simulink model "BaseEngineController_LS_128"  (Simulink 7.7)
settings: Solver=FixedStepDiscrete  StartTime=0.0  StopTime=10.0  RelTol=1e-3
PreLoadFcn:
  | try, eval([bdroot '_setup']); catch, eval('model_setup', ''); end
InitFcn:
  | try, eval([bdroot '_setup']); catch, eval('model_setup', ''); end
undefined symbols (not defined in the file): ECU565, High, motohawk_build_version, motohawk_trunc_name, motohawk_vardec_config_group, motohawk_vardec_path, True
libraries: MotoHawk_lib x1418, motohawk_control_primitives_lib x183, motohawk_engine_lib x32, simulink x21, motohawk_annotations_lib x9, AutoDoc_lib x8, simulink_extras x4, motohawk_ccp_examples_lib x1, motohawk_control_primitives_motoshare_lib x1
(part 23 of 27)

== system BaseEngineController_LS_128/Foreground/Control/Controller/Run/O2 Control/O2 PID Calibrations ==
  Sensors : Inport
  Bus Creator : BusCreator  Inputs=12
  Error Gain Scheduling : Subsystem
  O2 Control Switch Point Maps : Subsystem
  motohawk_calibration10 : MotoHawk_lib/Calibration & Probing Blocks/motohawk_calibration  nam='O2CtrlPIDOutUpperLimit'  val=10  storage=Calibration  show_more=on  name_source=Use Parameter  data_type=Inherit from 'Default Value'  read_level=1  write_level=1  ovr_cals=on  view_as=Number  enum_struct={'Disabled', 'Enabled'}  vector_style=Wide Row  use_help_units=on  help='Upper limit on gaseous closed loop O2 PID Output.'  units='mult'  use_header_enum=off  row_header_enum={}  col_header_enum={}  use_min_max=off  min_val=-inf  max_val=inf  use_precision=off  precision='5.3'  gain=1  offset=0  exp=1  use_mototune_group=on  mototune_group=motohawk_vardec_path(gcb)
  motohawk_calibration11 : MotoHawk_lib/Calibration & Probing Blocks/motohawk_calibration  nam='O2CtrlPIDOutLowerLimit'  val=-10  storage=Calibration  show_more=on  name_source=Use Parameter  data_type=Inherit from 'Default Value'  read_level=1  write_level=1  ovr_cals=on  view_as=Number  enum_struct={'Disabled', 'Enabled'}  vector_style=Wide Row  use_help_units=on  help='Lower limit on gaseous closed loop O2 PID Output.'  units='mult'  use_header_enum=off  row_header_enum={}  col_header_enum={}  use_min_max=off  min_val=-inf  max_val=inf  use_precision=off  precision='5.3'  gain=1  offset=0  exp=1  use_mototune_group=on  mototune_group=motohawk_vardec_path(gcb)
  motohawk_calibration5 : MotoHawk_lib/Calibration & Probing Blocks/motohawk_calibration  nam='O2CtrlPGain'  val=1  storage=Calibration  show_more=on  name_source=Use Parameter  data_type=Inherit from 'Default Value'  read_level=1  write_level=1  ovr_cals=on  view_as=Number  enum_struct={'Disabled', 'Enabled'}  vector_style=Wide Row  use_help_units=on  help='Base P-gain for the gaseous closed loop O2 controller.'  units='mult'  use_header_enum=off  row_header_enum={}  col_header_enum={}  use_min_max=off  min_val=-inf  max_val=inf  use_precision=off  precision='5.3'  gain=1  offset=0  exp=1  use_mototune_group=on  mototune_group=motohawk_vardec_path(gcb)
  motohawk_calibration6 : MotoHawk_lib/Calibration & Probing Blocks/motohawk_calibration  nam='O2CtrlIGain'  val=1  storage=Calibration  show_more=on  name_source=Use Parameter  data_type=Inherit from 'Default Value'  read_level=1  write_level=1  ovr_cals=on  view_as=Number  enum_struct={'Disabled', 'Enabled'}  vector_style=Wide Row  use_help_units=on  help='Base I-gain for the gaseous closed loop O2 controller.'  units='mult'  use_header_enum=off  row_header_enum={}  col_header_enum={}  use_min_max=off  min_val=-inf  max_val=inf  use_precision=off  precision='5.3'  gain=1  offset=0  exp=1  use_mototune_group=on  mototune_group=motohawk_vardec_path(gcb)
  motohawk_calibration7 : MotoHawk_lib/Calibration & Probing Blocks/motohawk_calibration  nam='O2CtrlDGain'  val=0.5  storage=Calibration  show_more=on  name_source=Use Parameter  data_type=Inherit from 'Default Value'  read_level=1  write_level=1  ovr_cals=on  view_as=Number  enum_struct={'Disabled', 'Enabled'}  vector_style=Wide Row  use_help_units=on  help='Base D-gain for the gaseous closed loop O2 controller.'  units='mult'  use_header_enum=off  row_header_enum={}  col_header_enum={}  use_min_max=off  min_val=-inf  max_val=inf  use_precision=off  precision='5.3'  gain=1  offset=0  exp=1  use_mototune_group=on  mototune_group=motohawk_vardec_path(gcb)
  motohawk_calibration8 : MotoHawk_lib/Calibration & Probing Blocks/motohawk_calibration  nam='O2ITermLowerLimit'  val=-0.5  storage=Calibration  show_more=on  name_source=Use Parameter  data_type=Inherit from 'Default Value'  read_level=1  write_level=1  ovr_cals=on  view_as=Number  enum_struct={'Disabled', 'Enabled'}  vector_style=Wide Row  use_help_units=on  help='Lower limit on gaseous closed loop O2 I Term.'  units='mult'  use_header_enum=off  row_header_enum={}  col_header_enum={}  use_min_max=off  min_val=-inf  max_val=inf  use_precision=off  precision='5.3'  gain=1  offset=0  exp=1  use_mototune_group=on  mototune_group=motohawk_vardec_path(gcb)
  motohawk_calibration9 : MotoHawk_lib/Calibration & Probing Blocks/motohawk_calibration  nam='O2ITermUpperLimit'  val=0.5  storage=Calibration  show_more=on  name_source=Use Parameter  data_type=Inherit from 'Default Value'  read_level=1  write_level=1  ovr_cals=on  view_as=Number  enum_struct={'Disabled', 'Enabled'}  vector_style=Wide Row  use_help_units=on  help='Upper limit on gaseous closed loop O2 I Term.'  units='mult'  use_header_enum=off  row_header_enum={}  col_header_enum={}  use_min_max=off  min_val=-inf  max_val=inf  use_precision=off  precision='5.3'  gain=1  offset=0  exp=1  use_mototune_group=on  mototune_group=motohawk_vardec_path(gcb)
  Calibrations : Outport
  wires:
  O2 Control Switch Point Maps/1(RichTargetDelta) -> Bus Creator/1
  O2 Control Switch Point Maps/2(LeanTargetDelta) -> Bus Creator/2
  O2 Control Switch Point Maps/3(RichSwPtDelta) -> Bus Creator/3
  O2 Control Switch Point Maps/4(LeanSwPtDelta) -> Bus Creator/4
  Error Gain Scheduling/1(ErrorGain) -> Bus Creator/5  "O2ControlErrorGain"
  motohawk_calibration5/1 -> Bus Creator/6  "O2ControlPGain"
  motohawk_calibration6/1 -> Bus Creator/7  "O2ControlIGain"
  motohawk_calibration7/1 -> Bus Creator/8  "O2ControlDGain"
  motohawk_calibration9/1 -> Bus Creator/9  "O2ControlITermUpperLimit"
  motohawk_calibration8/1 -> Bus Creator/10  "O2ControlItermLowerLimit"
  motohawk_calibration10/1 -> Bus Creator/11  "O2ControlOutUpperLimit"
  motohawk_calibration11/1 -> Bus Creator/12  "O2ControlOutLowerLimit"
  Bus Creator/1 -> Calibrations/1
  Sensors/1 -> O2 Control Switch Point Maps/1(Sensors), Error Gain Scheduling/1(Sensors)

== system BaseEngineController_LS_128/Foreground/Control/Controller/Run/O2 Control/O2 PID Controller Bank A ==
  Hold PID : Inport
  O2Sensor : Inport  Port=2
  DesEquivRatio : Inport  Port=3
  Calibrations : Inport  Port=4
  Reset : Inport  Port=5
  Bus Selector : BusSelector  OutputSignals=RichEquivRatioTargetDelta,LeanEquivRatioTargetDelta,RichEquivRatioSwPtDelta,LeanEquivRatioSwPtDelta
  Bus Selector1 : BusSelector  OutputSignals=O2ControlErrorGain,O2ControlPGain,O2ControlIGain,O2ControlDGain,O2ControlITermUpperLimit,O2ControlItermLowerLimit,O2ControlOutUpperLimit,O2ControlOutLowerLimit
  Closed-Loop O2 PID Controller : Subsystem
  Equivalence Ratio Perturbation : Subsystem  Description=|
      | /* Name: PosPertMagnitude Unit:phi ClassID:VAR StorageID:FLASH Access:RW4+RW3+NA2+NA1 TypeID:UINT1               
      |    Gain:0.01 Min:0.00 Max:2.55 Format:5.2 UpdateID:REMOTE Group:"Engine Control | Run | Fuel | O2 Control | O2 " 
      |    "Control Config" Help:"Positive value added to EquivRatioWU for PosPertPeriod ms during the positive portion "
      |    "of the perturbation cycle. Used for catalyst efficiency optimization." VardecSig:6C */                       
      |                                                                                                                  
      | /* Name: NegPertMagnitude Unit:phi ClassID:VAR StorageID:FLASH Access:RW4+RW3+NA2+NA1 TypeID:UINT1               
      |    Gain:0.01 Min:0.00 Max:2.55 Format:5.2 UpdateID:REMOTE Group:"Engine Control | Run | Fuel | O2 Control | O2 " 
      |    "Control Config" Help:"Negative value added to EquivRatioWU for NegPertPeriod ms during the negative portion "
      |    "of the perturbation cycle. Used for catalyst efficiency optimization." VardecSig:6C */                       
      |                                                                                                                  
      | /* Name: PosPertPeriod Unit:ms ClassID:VAR StorageID:FLASH Access:RW4+RW3+NA2+NA1 TypeID:UINT1 Gain:5            
      |    Min:0.00 Max:1275.00 Format:5.2 UpdateID:REMOTE Group:"Engine Control | Run | Fuel | O2 Control | O2 "        
      |    "Control Config" Help:"Duration of the positive portion of the perturbation cycle. Used for catalyst "        
      |    "efficiency optimization." VardecSig:6C */                                                                    
      |                                                                                                                  
      | /* Name: NegPertPeriod Unit:ms ClassID:VAR StorageID:FLASH Access:RW4+RW3+NA2+NA1 TypeID:UINT1 Gain:5            
      |    Min:0.00 Max:1275.00 Format:5.2 UpdateID:REMOTE Group:"Engine Control | Run | Fuel | O2 Control | O2 "        
      |    "Control Config" Help:"Duration of the negative portion of the perturbation cycle. Used for catalyst "        
      |    "efficiency optimization." VardecSig:6C */
  Multiply by 1.0 if not yet enabled : InitialCondition  Value=1.0
  Switch : Switch  Threshold=1
  motohawk_probe : MotoHawk_lib/Calibration & Probing Blocks/motohawk_probe  nam='O2TargetEquivRatio_BankA'  show_more=on  name_source=Use Parameter  read_level=1  view_as=Number  enum_struct={'Disabled', 'Enabled'}  vector_style=Wide Row  use_help_units=on  help='Current target equivalence ratio for closed-loop O2 control.'  units='ratio'  use_header_enum=off  row_header_enum={}  col_header_enum={}  use_precision=off  precision=''  gain=1  offset=0  exp=1  use_mototune_group=on  mototune_group=motohawk_vardec_path(gcb)
  FuelMult : Outport  InitialOutput=1
  O2 Error : Outport  Port=2  InitialOutput=0
  wires:
  Reset/1 -> Closed-Loop O2 PID Controller/11(Reset), Equivalence Ratio Perturbation/8(RunStateDisabled)
  Equivalence Ratio Perturbation/1(Target Phi) -> Switch/3
  Switch/1 -> motohawk_probe/1, Closed-Loop O2 PID Controller/2(TargetEquivRatio)
  Hold PID/1 -> Switch/2, Equivalence Ratio Perturbation/7(O2Disabled)
  O2Sensor/1 -> Switch/1, Closed-Loop O2 PID Controller/1(O2Sensor), Equivalence Ratio Perturbation/1(O2Sensor)
  Closed-Loop O2 PID Controller/1(Multiplier) -> Multiply by 1.0 if not yet enabled/1
  DesEquivRatio/1 -> Equivalence Ratio Perturbation/2(DesEquivRatio)
  Calibrations/1 -> Bus Selector/1, Bus Selector1/1
  Bus Selector/1 -> Equivalence Ratio Perturbation/3(RichEquivRatioTargetDelta)  "<RichEquivRatioTargetDelta>"
  Bus Selector/2 -> Equivalence Ratio Perturbation/4(LeanEquivRatioTargetDelta)  "<LeanEquivRatioTargetDelta>"
  Bus Selector/3 -> Equivalence Ratio Perturbation/5(RichEquivRatioSwPtDelta)  "<RichEquivRatioSwPtDelta>"
  Bus Selector/4 -> Equivalence Ratio Perturbation/6(LeanEquivRatioSwPtDelta)  "<LeanEquivRatioSwPtDelta>"
  Bus Selector1/1 -> Closed-Loop O2 PID Controller/3(ErrorGain)  "<O2ControlErrorGain>"
  Bus Selector1/2 -> Closed-Loop O2 PID Controller/4(PGain)  "<O2ControlPGain>"
  Bus Selector1/3 -> Closed-Loop O2 PID Controller/5(IGain)  "<O2ControlIGain>"
  Bus Selector1/4 -> Closed-Loop O2 PID Controller/6(DGain)  "<O2ControlDGain>"
  Bus Selector1/5 -> Closed-Loop O2 PID Controller/7(ITermUpperLimit)  "<O2ControlITermUpperLimit>"
  Bus Selector1/6 -> Closed-Loop O2 PID Controller/8(ITermLowerLimit)  "<O2ControlItermLowerLimit>"
  Bus Selector1/7 -> Closed-Loop O2 PID Controller/9(OutUpperLimit)  "<O2ControlOutUpperLimit>"
  Bus Selector1/8 -> Closed-Loop O2 PID Controller/10(OutLowerLimit)  "<O2ControlOutLowerLimit>"
  Multiply by 1.0 if not yet enabled/1 -> FuelMult/1
  Closed-Loop O2 PID Controller/2(ITerm) -> O2 Error/1

== system BaseEngineController_LS_128/Foreground/Control/Controller/Run/O2 Control/O2 PID Controller Bank B ==
  Hold PID : Inport
  O2Sensor : Inport  Port=2
  DesEquivRatio : Inport  Port=3
  Calibrations : Inport  Port=4
  Reset : Inport  Port=5
  Bus Selector : BusSelector  OutputSignals=RichEquivRatioTargetDelta,LeanEquivRatioTargetDelta,RichEquivRatioSwPtDelta,LeanEquivRatioSwPtDelta
  Bus Selector1 : BusSelector  OutputSignals=O2ControlErrorGain,O2ControlPGain,O2ControlIGain,O2ControlDGain,O2ControlITermUpperLimit,O2ControlItermLowerLimit,O2ControlOutUpperLimit,O2ControlOutLowerLimit
  Closed-Loop O2 PID Controller : Subsystem
  Equivalence Ratio Perturbation : Subsystem  Description=|
      | /* Name: PosPertMagnitude Unit:phi ClassID:VAR StorageID:FLASH Access:RW4+RW3+NA2+NA1 TypeID:UINT1               
      |    Gain:0.01 Min:0.00 Max:2.55 Format:5.2 UpdateID:REMOTE Group:"Engine Control | Run | Fuel | O2 Control | O2 " 
      |    "Control Config" Help:"Positive value added to EquivRatioWU for PosPertPeriod ms during the positive portion "
      |    "of the perturbation cycle. Used for catalyst efficiency optimization." VardecSig:6C */                       
      |                                                                                                                  
      | /* Name: NegPertMagnitude Unit:phi ClassID:VAR StorageID:FLASH Access:RW4+RW3+NA2+NA1 TypeID:UINT1               
      |    Gain:0.01 Min:0.00 Max:2.55 Format:5.2 UpdateID:REMOTE Group:"Engine Control | Run | Fuel | O2 Control | O2 " 
      |    "Control Config" Help:"Negative value added to EquivRatioWU for NegPertPeriod ms during the negative portion "
      |    "of the perturbation cycle. Used for catalyst efficiency optimization." VardecSig:6C */                       
      |                                                                                                                  
      | /* Name: PosPertPeriod Unit:ms ClassID:VAR StorageID:FLASH Access:RW4+RW3+NA2+NA1 TypeID:UINT1 Gain:5            
      |    Min:0.00 Max:1275.00 Format:5.2 UpdateID:REMOTE Group:"Engine Control | Run | Fuel | O2 Control | O2 "        
      |    "Control Config" Help:"Duration of the positive portion of the perturbation cycle. Used for catalyst "        
      |    "efficiency optimization." VardecSig:6C */                                                                    
      |                                                                                                                  
      | /* Name: NegPertPeriod Unit:ms ClassID:VAR StorageID:FLASH Access:RW4+RW3+NA2+NA1 TypeID:UINT1 Gain:5            
      |    Min:0.00 Max:1275.00 Format:5.2 UpdateID:REMOTE Group:"Engine Control | Run | Fuel | O2 Control | O2 "        
      |    "Control Config" Help:"Duration of the negative portion of the perturbation cycle. Used for catalyst "        
      |    "efficiency optimization." VardecSig:6C */
  Multiply by 1.0 if not yet enabled : InitialCondition  Value=1.0
  Switch : Switch  Threshold=1
  motohawk_probe : MotoHawk_lib/Calibration & Probing Blocks/motohawk_probe  nam='O2TargetEquivRatio_BankB'  show_more=on  name_source=Use Parameter  read_level=1  view_as=Number  enum_struct={'Disabled', 'Enabled'}  vector_style=Wide Row  use_help_units=on  help='Current target equivalence ratio for closed-loop O2 control.'  units='ratio'  use_header_enum=off  row_header_enum={}  col_header_enum={}  use_precision=off  precision=''  gain=1  offset=0  exp=1  use_mototune_group=on  mototune_group=motohawk_vardec_path(gcb)
  FuelMult : Outport  InitialOutput=1
  O2 Error : Outport  Port=2  InitialOutput=0
  wires:
  Reset/1 -> Closed-Loop O2 PID Controller/11(Reset), Equivalence Ratio Perturbation/8(RunStateDisabled)
  Equivalence Ratio Perturbation/1(Target Phi) -> Switch/3
  Switch/1 -> motohawk_probe/1, Closed-Loop O2 PID Controller/2(TargetEquivRatio)
  Hold PID/1 -> Switch/2, Equivalence Ratio Perturbation/7(O2Disabled)
  O2Sensor/1 -> Switch/1, Closed-Loop O2 PID Controller/1(O2Sensor), Equivalence Ratio Perturbation/1(O2Sensor)
  Closed-Loop O2 PID Controller/1(Multiplier) -> Multiply by 1.0 if not yet enabled/1
  DesEquivRatio/1 -> Equivalence Ratio Perturbation/2(DesEquivRatio)
  Calibrations/1 -> Bus Selector/1, Bus Selector1/1
  Bus Selector/1 -> Equivalence Ratio Perturbation/3(RichEquivRatioTargetDelta)  "<RichEquivRatioTargetDelta>"
  Bus Selector/2 -> Equivalence Ratio Perturbation/4(LeanEquivRatioTargetDelta)  "<LeanEquivRatioTargetDelta>"
  Bus Selector/3 -> Equivalence Ratio Perturbation/5(RichEquivRatioSwPtDelta)  "<RichEquivRatioSwPtDelta>"
  Bus Selector/4 -> Equivalence Ratio Perturbation/6(LeanEquivRatioSwPtDelta)  "<LeanEquivRatioSwPtDelta>"
  Bus Selector1/1 -> Closed-Loop O2 PID Controller/3(ErrorGain)  "<O2ControlErrorGain>"
  Bus Selector1/2 -> Closed-Loop O2 PID Controller/4(PGain)  "<O2ControlPGain>"
  Bus Selector1/3 -> Closed-Loop O2 PID Controller/5(IGain)  "<O2ControlIGain>"
  Bus Selector1/4 -> Closed-Loop O2 PID Controller/6(DGain)  "<O2ControlDGain>"
  Bus Selector1/5 -> Closed-Loop O2 PID Controller/7(ITermUpperLimit)  "<O2ControlITermUpperLimit>"
  Bus Selector1/6 -> Closed-Loop O2 PID Controller/8(ITermLowerLimit)  "<O2ControlItermLowerLimit>"
  Bus Selector1/7 -> Closed-Loop O2 PID Controller/9(OutUpperLimit)  "<O2ControlOutUpperLimit>"
  Bus Selector1/8 -> Closed-Loop O2 PID Controller/10(OutLowerLimit)  "<O2ControlOutLowerLimit>"
  Multiply by 1.0 if not yet enabled/1 -> FuelMult/1
  Closed-Loop O2 PID Controller/2(ITerm) -> O2 Error/1

== system BaseEngineController_LS_128/Foreground/Control/Controller/Run/O2 Control/O2Arb ==
  BankEnable : Inport
  O2PidOut : Inport  Port=2
  Constant : Constant
  Switch : Switch  Threshold=1
  motohawk_probe4 : MotoHawk_lib/Calibration & Probing Blocks/motohawk_probe  nam='O2FuelMult'  show_more=on  name_source=Use Parameter  read_level=1  view_as=Number  enum_struct={'Disabled', 'Enabled'}  vector_style=Wide Row  use_help_units=on  help='Closed-loop O2 control fuel multiplier.'  units='mult'  use_header_enum=off  row_header_enum={}  col_header_enum={}  use_precision=off  precision=''  gain=1  offset=0  exp=1  use_mototune_group=on  mototune_group=motohawk_vardec_path(gcb)
  FuelMult : Outport
  wires:
  O2PidOut/1 -> Switch/1  "O2FuelMult"
  Constant/1 -> Switch/3
  BankEnable/1 -> Switch/2
  Switch/1 -> FuelMult/1, motohawk_probe4/1  "O2FuelMult"

== system BaseEngineController_LS_128/Foreground/Control/Controller/Run/O2 Control/O2Disable ==
  Bank1Valid : Inport
  Bank2Valid : Inport  Port=2
  Logical Operator : Logic  Operator=NOT  AllPortsSameDT=off  OutDataTypeStr=boolean
  Logical Operator1 : Logic  Operator=NOT  AllPortsSameDT=off  OutDataTypeStr=boolean
  Logical Operator2 : Logic  AllPortsSameDT=off  OutDataTypeStr=boolean
  Logical Operator3 : Logic  Operator=OR  Inputs=3  AllPortsSameDT=off  OutDataTypeStr=boolean
  motohawk_calibration : MotoHawk_lib/Calibration & Probing Blocks/motohawk_calibration  nam='BankB_Enbl'  val=1  storage=Calibration  show_more=on  name_source=Use Parameter  data_type=boolean  read_level=1  write_level=1  ovr_cals=on  view_as=Enumeration  enum_struct={'Disabled', 'Enabled'}  vector_style=Wide Row  use_help_units=off  help=''  units=''  use_header_enum=off  row_header_enum={}  col_header_enum={}  use_min_max=off  min_val=-inf  max_val=inf  use_precision=off  precision=''  gain=1  offset=0  exp=1  use_mototune_group=off  mototune_group=motohawk_vardec_path(gcb)
  motohawk_fault_action : MotoHawk_lib/Fault Management Blocks/motohawk_fault_action  nam='DisableO2Ctrl'  output_status=on  eval_nam=DisableO2Ctrl
  motohawk_probe : MotoHawk_lib/Calibration & Probing Blocks/motohawk_probe  nam='O2FaultDisable'  show_more=off  name_source=Use Parameter  read_level=1  view_as=Number  enum_struct={'Disabled', 'Enabled'}  vector_style=Wide Row  use_help_units=off  help=''  units=''  use_header_enum=off  row_header_enum={}  col_header_enum={}  use_precision=off  precision=''  gain=1  offset=0  exp=1  use_mototune_group=off  mototune_group=motohawk_vardec_path(gcb)
  Out1 : Outport
  wires:
  Bank1Valid/1 -> Logical Operator/1
  Bank2Valid/1 -> Logical Operator1/1
  Logical Operator1/1 -> Logical Operator2/1
  Logical Operator/1 -> Logical Operator3/1
  Logical Operator2/1 -> Logical Operator3/2
  motohawk_fault_action/1 -> Logical Operator3/3
  Logical Operator3/1 -> Out1/1, motohawk_probe/1
  motohawk_calibration/1 -> Logical Operator2/2

== system BaseEngineController_LS_128/Foreground/Control/Controller/Run/Spark Manager/Desired Eq Ratio Offset ==
  Sensors : Inport
  DesiredEqRatio : Inport  Port=2
  Bus Selector : BusSelector  OutputSignals=RawIndexes.MAP09Idx,RawIndexes.RPM09Idx
  Product : Product  RndMeth=Zero
  motohawk_interpolation_1d : MotoHawk_lib/Lookup Tables/motohawk_interpolation_1d  nam='EqRatio_SpkOfst'  table_data=zeros(1,9)  show_more=on  data_type=Inherit from 'Table Data'  storage=NonAdaptive  read_level=1  write_level=1  ovr_cals=on  use_help=on  help='Spark offset based on desired equivalence ratio (also muliplied by a speed load factor)'  units='degCA'  use_min_max=off  min_val=-inf  max_val=inf  use_precision=off  precision=''  gain=1  offset=0  exp=1  use_links=on  prelookup_block='DesEqRatio09'  output_name=''  use_mototune_group=on  mototune_group=motohawk_vardec_path(gcb)
  motohawk_interpolation_2d3 : MotoHawk_lib/Lookup Tables/motohawk_interpolation_2d  nam='EqRatio_SpkOfsMult'  table_data=ones(9)  show_more=on  data_type=Inherit from 'Table Data'  storage=NonAdaptive  read_level=1  write_level=1  ovr_cals=on  use_help=on  help='Speed and Load Multiplier to the Equivalence Ratio Spark Offset table.'  units='mult'  use_min_max=off  min_val=-inf  max_val=inf  use_precision=on  precision=''  gain=1  offset=0  exp=1  use_links=on  row_prelookup_block=''  col_prelookup_block=''  output_name=''  use_mototune_group=on  mototune_group=motohawk_vardec_path(gcb)
  motohawk_prelookup : MotoHawk_lib/Lookup Tables/motohawk_prelookup  nam='DesEqRatio09'  breakpoint_data=[0 0.1 0.2 0.3 0.4 0.45 0.5 0.6 0.9]  show_more=on  data_type=Inherit from 'Table Data'  storage=Constant  read_level=1  write_level=1  ovr_cals=on  use_help=on  help='Desired Equivalence Ratio breakpoints'  units='F/A'  use_min_max=off  min_val=0  max_val=inf  use_precision=off  precision=''  gain=1  offset=0  exp=1  use_links=on  input_name=''  use_mototune_group=on  mototune_group=motohawk_vardec_path(gcb)
  motohawk_probe : MotoHawk_lib/Calibration & Probing Blocks/motohawk_probe  nam='Tot_EqRatio_SpkOfst'  show_more=on  name_source=Use Parameter  read_level=1  view_as=Number  enum_struct={'Disabled', 'Enabled'}  vector_style=Wide Row  use_help_units=on  help='Total Spark Offset based on Desired Equivalence Ratio, engine speed and load'  units='degCA'  use_header_enum=off  row_header_enum={}  col_header_enum={}  use_precision=off  precision=''  gain=1  offset=0  exp=1  use_mototune_group=on  mototune_group=motohawk_vardec_path(gcb)
  EqRatioSpkOfst : Outport
  wires:
  Bus Selector/2 -> motohawk_interpolation_2d3/2  "<RPM09Idx>"
  Bus Selector/1 -> motohawk_interpolation_2d3/1  "<MAP09Idx>"
  motohawk_interpolation_1d/1 -> Product/1
  Product/1 -> EqRatioSpkOfst/1, motohawk_probe/1
  Sensors/1 -> Bus Selector/1
  motohawk_prelookup/1 -> motohawk_interpolation_1d/1
  DesiredEqRatio/1 -> motohawk_prelookup/1
  motohawk_interpolation_2d3/1 -> Product/2  "RichEquivRatioTargetDelta"

== system BaseEngineController_LS_128/Foreground/Control/Controller/Run/Spark Manager/Ethanol Spark Offset ==
  Sensors : Inport
  Bus Selector : BusSelector  OutputSignals=RawIndexes.MAP09Idx,RawIndexes.RPM09Idx
  Bus Selector3 : BusSelector  OutputSignals=RawIndexes.OXY05Idx
  Product : Product  RndMeth=Zero
  motohawk_interpolation_1d : MotoHawk_lib/Lookup Tables/motohawk_interpolation_1d  nam='EthSpkMod'  table_data=[0,0,0,0,0]  show_more=on  data_type=Inherit from 'Table Data'  storage=NonAdaptive  read_level=1  write_level=1  ovr_cals=on  use_help=on  help='Spark advance as a function of ethanol %'  units='degBTDC'  use_min_max=off  min_val=-inf  max_val=inf  use_precision=off  precision=''  gain=1  offset=0  exp=1  use_links=off  prelookup_block=''  output_name=''  use_mototune_group=off  mototune_group=motohawk_vardec_path(gcb)
  motohawk_interpolation_2d3 : MotoHawk_lib/Lookup Tables/motohawk_interpolation_2d  nam='Ethanol_SpkOfstMult'  table_data=ones(9)  show_more=on  data_type=Inherit from 'Table Data'  storage=NonAdaptive  read_level=1  write_level=1  ovr_cals=on  use_help=on  help='Multiplier on ECT spark offset table.'  units='mult'  use_min_max=off  min_val=-inf  max_val=inf  use_precision=on  precision=''  gain=1  offset=0  exp=1  use_links=off  row_prelookup_block=''  col_prelookup_block=''  output_name=''  use_mototune_group=on  mototune_group=motohawk_vardec_path(gcb)
  motohawk_probe : MotoHawk_lib/Calibration & Probing Blocks/motohawk_probe  nam='Ethanol_Spk_Ofst'  show_more=on  name_source=Use Parameter  read_level=1  view_as=Number  enum_struct={'Disabled', 'Enabled'}  vector_style=Wide Row  use_help_units=on  help='Total Spark Offset based on ECT, IAT2, engine speed and load'  units='degCA'  use_header_enum=off  row_header_enum={}  col_header_enum={}  use_precision=off  precision=''  gain=1  offset=0  exp=1  use_mototune_group=on  mototune_group=motohawk_vardec_path(gcb)
  EthanolSpkOfst : Outport
  wires:
  Sensors/1 -> Bus Selector3/1, Bus Selector/1
  Bus Selector3/1 -> motohawk_interpolation_1d/1  "<OXY05Idx>"
  Bus Selector/1 -> motohawk_interpolation_2d3/1  "<MAP09Idx>"
  motohawk_interpolation_2d3/1 -> Product/2  "RichEquivRatioTargetDelta"
  Bus Selector/2 -> motohawk_interpolation_2d3/2  "<RPM09Idx>"
  motohawk_interpolation_1d/1 -> Product/1
  Product/1 -> EthanolSpkOfst/1, motohawk_probe/1

== system BaseEngineController_LS_128/Foreground/Control/Controller/Run/Spark Manager/Spark Advance Rate Limiter ==
  DesSparkAdv : Inport
  First Time : motohawk_control_primitives_lib/First Time  SystemSampleTime=-1
  Saturation : motohawk_control_primitives_lib/Saturation  SystemSampleTime=-1
  Sum : Sum  Inputs=|++  SaturateOnIntegerOverflow=on
  Sum1 : Sum  Inputs=-+|  SaturateOnIntegerOverflow=on
  Switch : Switch  Threshold=1  OutDataTypeStr=Inherit: Inherit via back propagation  SaturateOnIntegerOverflow=on  InputSameDT=on
  Unit Delay : UnitDelay  SampleTime=-1
  motohawk_calibration : MotoHawk_lib/Calibration & Probing Blocks/motohawk_calibration  nam='SparkAdv_DeltaHi'  val=5  storage=Calibration  show_more=on  name_source=Use Parameter  data_type=Inherit from 'Default Value'  read_level=1  write_level=1  ovr_cals=on  view_as=Number  enum_struct={'Disabled', 'Enabled'}  vector_style=Wide Row  use_help_units=on  help='Maximum increasing spark change per 5ms'  units='degCA'  use_header_enum=off  row_header_enum={}  col_header_enum={}  use_min_max=on  min_val=0  max_val=720  use_precision=off  precision=''  gain=1  offset=0  exp=1  use_mototune_group=on  mototune_group=motohawk_vardec_path(gcb)
  motohawk_calibration1 : MotoHawk_lib/Calibration & Probing Blocks/motohawk_calibration  nam='SparkAdv_DeltaLo'  val=5  storage=Calibration  show_more=on  name_source=Use Parameter  data_type=Inherit from 'Default Value'  read_level=1  write_level=1  ovr_cals=on  view_as=Number  enum_struct={'Disabled', 'Enabled'}  vector_style=Wide Row  use_help_units=on  help='Maximum decreasing spark change per 5ms'  units='degBTDC'  use_header_enum=off  row_header_enum={}  col_header_enum={}  use_min_max=on  min_val=0  max_val=720  use_precision=off  precision=''  gain=1  offset=0  exp=1  use_mototune_group=on  mototune_group=motohawk_vardec_path(gcb)
  SparkAdv : Outport
  wires:
  DesSparkAdv/1 -> Saturation/1, Switch/1
  Sum1/1 -> Saturation/2
  Sum/1 -> Saturation/3
  Switch/1 -> Unit Delay/1, SparkAdv/1
  Saturation/1 -> Switch/3
  Unit Delay/1 -> Sum1/2, Sum/1
  First Time/1 -> Switch/2
  motohawk_calibration/1 -> Sum/2
  motohawk_calibration1/1 -> Sum1/1

== system BaseEngineController_LS_128/Foreground/Control/Controller/Run/Spark Manager/SparkAdvanceLimiter ==
  DesSparkAdv : Inport
  OnIdle : Inport  Port=2
  Sensors : Inport  Port=3
  Bus Selector3 : BusSelector  OutputSignals=RawIndexes.MAP09Idx
  Saturation : motohawk_control_primitives_lib/Saturation  SystemSampleTime=-1
  Switch1 : Switch  Threshold=0.5
  motohawk_calibration1 : MotoHawk_lib/Calibration & Probing Blocks/motohawk_calibration  nam='MaxSparkLimitOffIdle'  val=36  storage=Calibration  show_more=on  name_source=Use Parameter  data_type=Inherit from 'Default Value'  read_level=1  write_level=1  ovr_cals=on  view_as=Number  enum_struct={'Disabled', 'Enabled'}  vector_style=Wide Row  use_help_units=on  help='Max. spark limit on the delivered spark advance, when not in idle control.'  units='degBTDC'  use_header_enum=off  row_header_enum={}  col_header_enum={}  use_min_max=off  min_val=-inf  max_val=inf  use_precision=off  precision=''  gain=1  offset=0  exp=1  use_mototune_group=on  mototune_group=motohawk_vardec_path(gcb)
  motohawk_calibration5 : MotoHawk_lib/Calibration & Probing Blocks/motohawk_calibration  nam='MinSparkLimit'  val=-12  storage=Calibration  show_more=on  name_source=Use Parameter  data_type=Inherit from 'Default Value'  read_level=1  write_level=1  ovr_cals=on  view_as=Number  enum_struct={'Disabled', 'Enabled'}  vector_style=Wide Row  use_help_units=on  help='Min. spark limit on the delivered spark advance.'  units='degBTDC'  use_header_enum=off  row_header_enum={}  col_header_enum={}  use_min_max=on  min_val=-inf  max_val=inf  use_precision=off  precision=''  gain=1  offset=0  exp=1  use_mototune_group=on  mototune_group=motohawk_vardec_path(gcb)
  motohawk_interpolation_1d4 : MotoHawk_lib/Lookup Tables/motohawk_interpolation_1d  nam='MaxSparkLimit'  table_data=[15 16 18 19 19 19 19 18 18]  show_more=on  data_type=Inherit from 'Table Data'  storage=NonAdaptive  read_level=1  write_level=1  ovr_cals=on  use_help=on  help='Maximum allowable spark advance.'  units='degBTDC'  use_min_max=on  min_val=-inf  max_val=inf  use_precision=on  precision=''  gain=1  offset=0  exp=1  use_links=off  prelookup_block=''  output_name=''  use_mototune_group=on  mototune_group=motohawk_vardec_path(gcb)
  motohawk_probe : MotoHawk_lib/Calibration & Probing Blocks/motohawk_probe  nam='TotalSparkAdv'  show_more=on  name_source=Use Parameter  read_level=1  view_as=Number  enum_struct={'Disabled', 'Enabled'}  vector_style=Wide Row  use_help_units=on  help=''  units=''  use_header_enum=off  row_header_enum={}  col_header_enum={}  use_precision=on  precision=''  gain=1  offset=0  exp=1  use_mototune_group=on  mototune_group=motohawk_vardec_path(gcb)
  SparkAdv : Outport
  wires:
  motohawk_calibration5/1 -> Saturation/2
  Sensors/1 -> Bus Selector3/1
  Bus Selector3/1 -> motohawk_interpolation_1d4/1  "<MAP09Idx>"
  Switch1/1 -> Saturation/3
  OnIdle/1 -> Switch1/2
  motohawk_interpolation_1d4/1 -> Switch1/1
  motohawk_calibration1/1 -> Switch1/3
  DesSparkAdv/1 -> Saturation/1, motohawk_probe/1
  Saturation/1 -> SparkAdv/1

== system BaseEngineController_LS_128/Foreground/Control/Controller/Run/Spark Manager/Temp Comp Offset ==
  Sensors : Inport
  Add : Sum  Inputs=+++
  Bus Selector : BusSelector  OutputSignals=RawIndexes.MAP09Idx,RawIndexes.RPM09Idx
  Bus Selector1 : BusSelector  OutputSignals=RawIndexes.IAT05Idx
  Bus Selector2 : BusSelector  OutputSignals=RawIndexes.MAP09Idx,RawIndexes.RPM09Idx
  Bus Selector3 : BusSelector  OutputSignals=RawIndexes.ECT05Idx
  Bus Selector4 : BusSelector  OutputSignals=RawIndexes.CAT05Idx
  Bus Selector5 : BusSelector  OutputSignals=RawIndexes.MAP09Idx,RawIndexes.RPM09Idx
  Product : Product  RndMeth=Zero
  Product1 : Product  RndMeth=Zero
  Product2 : Product  RndMeth=Zero
  motohawk_interpolation_1d : MotoHawk_lib/Lookup Tables/motohawk_interpolation_1d  nam='ECT_SpkOfst'  table_data=zeros(1,5)  show_more=on  data_type=Inherit from 'Table Data'  storage=NonAdaptive  read_level=1  write_level=1  ovr_cals=on  use_help=on  help='ECT spark offset'  units='degBTDC'  use_min_max=on  min_val=-50  max_val=50  use_precision=off  precision=''  gain=1  offset=0  exp=1  use_links=on  prelookup_block=''  output_name=''  use_mototune_group=on  mototune_group=motohawk_vardec_path(gcb)
  motohawk_interpolation_1d1 : MotoHawk_lib/Lookup Tables/motohawk_interpolation_1d  nam='IAT_SpkOfst'  table_data=zeros(1,5)  show_more=on  data_type=Inherit from 'Table Data'  storage=NonAdaptive  read_level=1  write_level=1  ovr_cals=on  use_help=on  help='IAT spark offset'  units='degBTDC'  use_min_max=on  min_val=-50  max_val=50  use_precision=off  precision=''  gain=1  offset=0  exp=1  use_links=off  prelookup_block=''  output_name=''  use_mototune_group=on  mototune_group=motohawk_vardec_path(gcb)
  motohawk_interpolation_1d2 : MotoHawk_lib/Lookup Tables/motohawk_interpolation_1d  nam='CAT_SpkOfst'  table_data=zeros(1,5)  show_more=on  data_type=Inherit from 'Table Data'  storage=NonAdaptive  read_level=1  write_level=1  ovr_cals=on  use_help=on  help='CAT spark offset'  units=''  use_min_max=on  min_val=-50  max_val=50  use_precision=off  precision=''  gain=1  offset=0  exp=1  use_links=off  prelookup_block=''  output_name=''  use_mototune_group=on  mototune_group=motohawk_vardec_path(gcb)
  motohawk_interpolation_2d1 : MotoHawk_lib/Lookup Tables/motohawk_interpolation_2d  nam='IAT_SpkOfstMult'  table_data=ones(9)  show_more=on  data_type=Inherit from 'Table Data'  storage=NonAdaptive  read_level=1  write_level=1  ovr_cals=on  use_help=on  help='Multiplier on IAT spark offset table.'  units=''  use_min_max=on  min_val=-100  max_val=100  use_precision=on  precision=''  gain=1  offset=0  exp=1  use_links=off  row_prelookup_block=''  col_prelookup_block=''  output_name=''  use_mototune_group=on  mototune_group=motohawk_vardec_path(gcb)
  motohawk_interpolation_2d2 : MotoHawk_lib/Lookup Tables/motohawk_interpolation_2d  nam='CAT_SpkOfstMult'  table_data=ones(9)  show_more=on  data_type=Inherit from 'Table Data'  storage=NonAdaptive  read_level=1  write_level=1  ovr_cals=on  use_help=on  help='Multiplier on IAT2 spark offset table.'  units='mult'  use_min_max=off  min_val=-inf  max_val=inf  use_precision=on  precision=''  gain=1  offset=0  exp=1  use_links=off  row_prelookup_block=''  col_prelookup_block=''  output_name=''  use_mototune_group=on  mototune_group=motohawk_vardec_path(gcb)
  motohawk_interpolation_2d3 : MotoHawk_lib/Lookup Tables/motohawk_interpolation_2d  nam='ECT_SpkOfstMult'  table_data=ones(9)  show_more=on  data_type=Inherit from 'Table Data'  storage=NonAdaptive  read_level=1  write_level=1  ovr_cals=on  use_help=on  help='Multiplier on ECT spark offset table.'  units=''  use_min_max=on  min_val=-100  max_val=100  use_precision=on  precision=''  gain=1  offset=0  exp=1  use_links=off  row_prelookup_block=''  col_prelookup_block=''  output_name=''  use_mototune_group=on  mototune_group=motohawk_vardec_path(gcb)
  motohawk_probe : MotoHawk_lib/Calibration & Probing Blocks/motohawk_probe  nam='SpkOfstTempFnl'  show_more=on  name_source=Use Parameter  read_level=1  view_as=Number  enum_struct={'Disabled', 'Enabled'}  vector_style=Wide Row  use_help_units=on  help='Total Spark Offset based on ECT, IAT, CAT, engine speed and load'  units='degBTDC'  use_header_enum=off  row_header_enum={}  col_header_enum={}  use_precision=off  precision=''  gain=1  offset=0  exp=1  use_mototune_group=on  mototune_group=motohawk_vardec_path(gcb)
  TempSpkOfst : Outport
  wires:
  Sensors/1 -> Bus Selector3/1, Bus Selector/1, Bus Selector1/1, Bus Selector2/1, Bus Selector4/1, Bus Selector5/1
  Add/1 -> TempSpkOfst/1, motohawk_probe/1
  Product/1 -> Add/1
  motohawk_interpolation_1d/1 -> Product/1
  motohawk_interpolation_1d1/1 -> Product1/1
  Product1/1 -> Add/2
  Bus Selector3/1 -> motohawk_interpolation_1d/1  "<ECT05Idx>"
  Bus Selector/1 -> motohawk_interpolation_2d3/1  "<MAP09Idx>"
  Bus Selector/2 -> motohawk_interpolation_2d3/2  "<RPM09Idx>"
  Bus Selector1/1 -> motohawk_interpolation_1d1/1  "<IAT05Idx>"
  Bus Selector2/1 -> motohawk_interpolation_2d1/1  "<MAP09Idx>"
  Bus Selector2/2 -> motohawk_interpolation_2d1/2  "<RPM09Idx>"
  motohawk_interpolation_2d3/1 -> Product/2  "RichEquivRatioTargetDelta"
  motohawk_interpolation_2d1/1 -> Product1/2  "RichEquivRatioTargetDelta"
  motohawk_interpolation_1d2/1 -> Product2/1
  Bus Selector4/1 -> motohawk_interpolation_1d2/1  "<CAT05Idx>"
  Bus Selector5/1 -> motohawk_interpolation_2d2/1  "<MAP09Idx>"
  Bus Selector5/2 -> motohawk_interpolation_2d2/2  "<RPM09Idx>"
  motohawk_interpolation_2d2/1 -> Product2/2  "RichEquivRatioTargetDelta"
  Product2/1 -> Add/3

== system BaseEngineController_LS_128/Foreground/Control/Controller/Stall/FAN Control/Hysterisis ==
  HiThresh : Inport
  LowThresh : Inport  Port=2
  Signal : Inport  Port=3
  Hysteresis : Subsystem
  LT : RelationalOperator  ZeroCross=off  InputSameDT=on
  LT1 : RelationalOperator  Operator=<=  ZeroCross=off  InputSameDT=on
  Threshold : Outport
  wires:
  LT/1 -> Hysteresis/1(Hi)  "AboveHiTarget"
  LT1/1 -> Hysteresis/2(Lo)  "BelowLoTarget"
  Signal/1 -> LT/1, LT1/1
  Hysteresis/1("Out (Lo=0, Hi=1)") -> Threshold/1
  HiThresh/1 -> LT/2
  LowThresh/1 -> LT1/2

== system BaseEngineController_LS_128/Foreground/Control/Controller/Stall/FAN Control/Hysterisis1 ==
  HiThresh : Inport
  LowThresh : Inport  Port=2
  Signal : Inport  Port=3
  Hysteresis : Subsystem
  LT : RelationalOperator  ZeroCross=off  InputSameDT=on
  LT1 : RelationalOperator  Operator=<=  ZeroCross=off  InputSameDT=on
  Threshold : Outport
  wires:
  LT/1 -> Hysteresis/1(Hi)  "AboveHiTarget"
  LT1/1 -> Hysteresis/2(Lo)  "BelowLoTarget"
  Signal/1 -> LT/1, LT1/1
  Hysteresis/1("Out (Lo=0, Hi=1)") -> Threshold/1
  HiThresh/1 -> LT/2
  LowThresh/1 -> LT1/2

== system BaseEngineController_LS_128/Foreground/Control/Controller/Stall/FAN Control/Hysterisis2 ==
  HiThresh : Inport
  LowThresh : Inport  Port=2
  Signal : Inport  Port=3
  Hysteresis : Subsystem
  LT : RelationalOperator  ZeroCross=off  InputSameDT=on
  LT1 : RelationalOperator  Operator=<=  ZeroCross=off  InputSameDT=on
  Threshold : Outport
  wires:
  LT/1 -> Hysteresis/1(Hi)  "AboveHiTarget"
  LT1/1 -> Hysteresis/2(Lo)  "BelowLoTarget"
  Signal/1 -> LT/1, LT1/1
  Hysteresis/1("Out (Lo=0, Hi=1)") -> Threshold/1
  HiThresh/1 -> LT/2
  LowThresh/1 -> LT1/2

== system BaseEngineController_LS_128/Foreground/Control/Diagnostics/MISFIRE/MisfireDiagSub/MisfireDiagFunc ==
  function : TriggerPort  TriggerType=function-call
  DetermineMisfire : Subsystem
  StoreRPMData : Subsystem

== system BaseEngineController_LS_128/Foreground/Control/VirtualSensors/AirCalcs/Capture Signal At Startup/Collect Average ==
  note: Collect samples by summing,
      | and divide by the total, to obtain average
  Count : Inport
  Signal : Inport  Port=2
  Enable : EnablePort  StatesWhenEnabling=reset
  Data Type Conversion : DataTypeConversion  SaturateOnIntegerOverflow=on  RndMeth=Zero
  Product : Product  Inputs=/*  OutDataTypeStr=Inherit: Same as first input
  Sum1 : Sum  Inputs=|++  InputSameDT=on
  Unit Delay1 : UnitDelay  SampleTime=-1
  Captured_Signal : Outport
  wires:
  Unit Delay1/1 -> Sum1/2
  Sum1/1 -> Unit Delay1/1, Product/2
  Signal/1 -> Sum1/1
  Product/1 -> Captured_Signal/1
  Count/1 -> Data Type Conversion/1
  Data Type Conversion/1 -> Product/1

== system BaseEngineController_LS_128/Foreground/Control/VirtualSensors/AirCalcs/Speed Density - MAP Referenced - Adaptive/Adapt VolEff Map ==
  MAFSens : Inport
  MAFSpdDensity : Inport  Port=2
  VE : Inport  Port=3
  Enable : EnablePort
  Add : Sum  Inputs=+-
  Divide : Product  Inputs=*/
  Divide1 : Product  Inputs=**
  Divide2 : Product  Inputs=**
  motohawk_adapt_table : MotoHawk_lib/Lookup Tables/motohawk_adapt_table  nam='VolEffAdaptMap'  typ=double  mode=Adapt between points  show_adapted=off
  motohawk_calibration : MotoHawk_lib/Calibration & Probing Blocks/motohawk_calibration  nam='VEAdaptMax'  val=false  storage=Calibration  show_more=on  name_source=Use Parameter  data_type=double  read_level=1  write_level=1  ovr_cals=on  view_as=Number  enum_struct={'Disabled', 'Enabled'}  vector_style=Wide Row  use_help_units=on  help='Determines whether the Volumetric Efficiency map will be adapted using the MAF sensor'  units='bool'  use_header_enum=off  row_header_enum={}  col_header_enum={}  use_min_max=off  min_val=-inf  max_val=inf  use_precision=off  precision=''  gain=1  offset=0  exp=1  use_mototune_group=on  mototune_group=motohawk_vardec_path(gcb)
  motohawk_calibration1 : MotoHawk_lib/Calibration & Probing Blocks/motohawk_calibration  nam='VEAdaptMin'  val=false  storage=Calibration  show_more=on  name_source=Use Parameter  data_type=double  read_level=1  write_level=1  ovr_cals=on  view_as=Number  enum_struct={'Disabled', 'Enabled'}  vector_style=Wide Row  use_help_units=on  help='Determines whether the Volumetric Efficiency map will be adapted using the MAF sensor'  units='bool'  use_header_enum=off  row_header_enum={}  col_header_enum={}  use_min_max=off  min_val=-inf  max_val=inf  use_precision=off  precision=''  gain=1  offset=0  exp=1  use_mototune_group=on  mototune_group=motohawk_vardec_path(gcb)
  motohawk_table_1d : MotoHawk_lib/Lookup Tables/motohawk_table_1d  SystemSampleTime=-1  nam='VEAdaptGainTbl'  bp_nam='VE_AdaptErrorIdxArr'  breakpoint_data=[1 2 3 4 5 6 7 8 9 10]  table_data=[1 2 3 4 5 6 7 8 9 10]  show_more=on  bp_data_type=Inherit from 'Breakpoint Data'  bp_storage=Constant  table_data_type=Inherit from 'Table Data'  storage=NonAdaptive  read_level=1  write_level=1  ovr_cals=on  use_help=on  help='Multiplier on error for adaptation, should always be positive'  bp_units=''  table_units=''  use_min_max=off  bp_min_val=-inf  bp_max_val=inf  min_val=-inf  max_val=inf  use_precision=off  use_breakpoint=off  b_precision=''  b_gain=1  b_offset=0  b_exp=1  use_table=off  t_precision=''  t_gain=1  t_offset=0  t_exp=1  use_links=off  input_name=''  output_name=''  use_mototune_group=on  mototune_group=motohawk_vardec_path(gcb)
  wires:
  motohawk_calibration1/1 -> motohawk_adapt_table/2
  motohawk_calibration/1 -> motohawk_adapt_table/3
  MAFSens/1 -> Add/1
  MAFSpdDensity/1 -> Add/2, Divide/2
  Add/1 -> Divide/1
  Divide/1 -> motohawk_table_1d/1, Divide2/2
  Divide1/1 -> motohawk_adapt_table/1
  motohawk_table_1d/1 -> Divide1/1
  VE/1 -> Divide2/1
  Divide2/1 -> Divide1/2

== system BaseEngineController_LS_128/Foreground/Control/VirtualSensors/AirCalcs/Speed Density - MAP Referenced - Adaptive/C to K1 ==
  C : Inport
  C to K : Fcn  Expr=u(1) + 273.2
  K : Outport
  wires:
  C to K/1 -> K/1
  C/1 -> C to K/1

== system BaseEngineController_LS_128/Foreground/Control/VirtualSensors/LoadBasedCalcs/Engine Steady-State Flag/Inc_DecFilterSelect1 ==
  In : Inport
  DecreasingFilter : Subsystem  TreatAsAtomicUnit=on
  First Order Low Pass : motohawk_control_primitives_lib/First Order Low Pass  SystemSampleTime=-1
  IncreasingFilter : Subsystem  TreatAsAtomicUnit=on
  Merge : Merge
  MinMax : MinMax  Function=max  Inputs=2  SaturateOnIntegerOverflow=on  InputSameDT=on
  Product : Product  Inputs=*/  SaturateOnIntegerOverflow=on  InputSameDT=on  OutDataTypeStr=Inherit: Same as first input
  Relational Operator3 : RelationalOperator  Operator=>  OutDataTypeStr=boolean
  Relational Operator4 : RelationalOperator  Operator=<  OutDataTypeStr=boolean
  Unit Delay{1..4} (4 alike) : UnitDelay  SampleTime=-1
  motohawk_delta_time : MotoHawk_lib/Extra Development Blocks/motohawk_delta_time  samp_time=.005  init_val=.005  mode=Seconds (double)
  motohawk_probe1 : MotoHawk_lib/Calibration & Probing Blocks/motohawk_probe  nam=[nam 'FilterConst']  show_more=on  name_source=Use Parameter  read_level=1  view_as=Number  enum_struct={'Disabled', 'Enabled'}  vector_style=Wide Row  use_help_units=off  help=''  units=''  use_header_enum=off  row_header_enum={}  col_header_enum={}  use_precision=off  precision=''  gain=1  offset=0  exp=1  use_mototune_group=on  mototune_group=grp_dis
  motohawk_probe2 : MotoHawk_lib/Calibration & Probing Blocks/motohawk_probe  nam=[nam 'Filtered']  show_more=on  name_source=Use Parameter  read_level=1  view_as=Number  enum_struct={'Disabled', 'Enabled'}  vector_style=Wide Row  use_help_units=off  help=''  units=''  use_header_enum=off  row_header_enum={}  col_header_enum={}  use_precision=off  precision=''  gain=1  offset=0  exp=1  use_mototune_group=on  mototune_group=grp_dis
  motohawk_probe3 : MotoHawk_lib/Calibration & Probing Blocks/motohawk_probe  nam=[nam 'Direction']  show_more=on  name_source=Use Parameter  read_level=1  view_as=Enumeration  enum_struct={'Decreasing', 'Increasing'}  vector_style=Wide Row  use_help_units=on  help=''  units=''  use_header_enum=off  row_header_enum={}  col_header_enum={}  use_precision=off  precision=''  gain=1  offset=0  exp=1  use_mototune_group=on  mototune_group=grp_dis
  Out : Outport
  wires:
  In/1 -> Relational Operator4/2, Relational Operator3/2, Unit Delay4/1, First Order Low Pass/1
  IncreasingFilter/1(Out1) -> Merge/1
  DecreasingFilter/1(Out1) -> Merge/2
  Relational Operator3/1 -> DecreasingFilter/Enable
  Relational Operator4/1 -> IncreasingFilter/Enable, motohawk_probe3/1
  Merge/1 -> motohawk_probe1/1, MinMax/2
  MinMax/1 -> Product/2
  motohawk_delta_time/1 -> Product/1, MinMax/1
  First Order Low Pass/1 -> motohawk_probe2/1, Out/1
  Product/1 -> First Order Low Pass/2
  Unit Delay2/1 -> Relational Operator3/1, Relational Operator4/1
  Unit Delay1/1 -> Unit Delay2/1
  Unit Delay3/1 -> Unit Delay1/1
  Unit Delay4/1 -> Unit Delay3/1

== system BaseEngineController_LS_128/Foreground/Control/VirtualSensors/LoadBasedCalcs/Engine Steady-State Flag/Inc_DecFilterSelect3 ==
  In : Inport
  DecreasingFilter : Subsystem  TreatAsAtomicUnit=on
  First Order Low Pass : motohawk_control_primitives_lib/First Order Low Pass  SystemSampleTime=-1
  IncreasingFilter : Subsystem  TreatAsAtomicUnit=on
  Merge : Merge
  MinMax : MinMax  Function=max  Inputs=2  SaturateOnIntegerOverflow=on  InputSameDT=on
  Product : Product  Inputs=*/  SaturateOnIntegerOverflow=on  InputSameDT=on  OutDataTypeStr=Inherit: Same as first input
  Relational Operator3 : RelationalOperator  Operator=>  OutDataTypeStr=boolean
  Relational Operator4 : RelationalOperator  Operator=<  OutDataTypeStr=boolean
  Unit Delay{1..4} (4 alike) : UnitDelay  SampleTime=-1
  motohawk_delta_time : MotoHawk_lib/Extra Development Blocks/motohawk_delta_time  samp_time=.005  init_val=.005  mode=Seconds (double)
  motohawk_probe1 : MotoHawk_lib/Calibration & Probing Blocks/motohawk_probe  nam=[nam 'FilterConst']  show_more=on  name_source=Use Parameter  read_level=1  view_as=Number  enum_struct={'Disabled', 'Enabled'}  vector_style=Wide Row  use_help_units=off  help=''  units=''  use_header_enum=off  row_header_enum={}  col_header_enum={}  use_precision=off  precision=''  gain=1  offset=0  exp=1  use_mototune_group=on  mototune_group=grp_dis
  motohawk_probe2 : MotoHawk_lib/Calibration & Probing Blocks/motohawk_probe  nam=[nam 'Filtered']  show_more=on  name_source=Use Parameter  read_level=1  view_as=Number  enum_struct={'Disabled', 'Enabled'}  vector_style=Wide Row  use_help_units=off  help=''  units=''  use_header_enum=off  row_header_enum={}  col_header_enum={}  use_precision=off  precision=''  gain=1  offset=0  exp=1  use_mototune_group=on  mototune_group=grp_dis
  motohawk_probe3 : MotoHawk_lib/Calibration & Probing Blocks/motohawk_probe  nam=[nam 'Direction']  show_more=on  name_source=Use Parameter  read_level=1  view_as=Enumeration  enum_struct={'Decreasing', 'Increasing'}  vector_style=Wide Row  use_help_units=on  help=''  units=''  use_header_enum=off  row_header_enum={}  col_header_enum={}  use_precision=off  precision=''  gain=1  offset=0  exp=1  use_mototune_group=on  mototune_group=grp_dis
  Out : Outport
  wires:
  In/1 -> Relational Operator4/2, Relational Operator3/2, Unit Delay4/1, First Order Low Pass/1
  IncreasingFilter/1(Out1) -> Merge/1
  DecreasingFilter/1(Out1) -> Merge/2
  Relational Operator3/1 -> DecreasingFilter/Enable
  Relational Operator4/1 -> IncreasingFilter/Enable, motohawk_probe3/1
  Merge/1 -> motohawk_probe1/1, MinMax/2
  MinMax/1 -> Product/2
  motohawk_delta_time/1 -> Product/1, MinMax/1
  First Order Low Pass/1 -> motohawk_probe2/1, Out/1
  Product/1 -> First Order Low Pass/2
  Unit Delay2/1 -> Relational Operator3/1, Relational Operator4/1
  Unit Delay1/1 -> Unit Delay2/1
  Unit Delay3/1 -> Unit Delay1/1
  Unit Delay4/1 -> Unit Delay3/1

== system BaseEngineController_LS_128/Foreground/Control/VirtualSensors/RawProcessed/Base TPS Request/PassThrough1 ==
  In1 : Inport
  Enable : EnablePort
  Out1 : Outport  InitialOutput=.005
  wires:
  In1/1 -> Out1/1

== system BaseEngineController_LS_128/Foreground/Control/VirtualSensors/RawProcessed/Base TPS Request/PassThrough2 ==
  In1 : Inport
  Enable : EnablePort
  Out1 : Outport  InitialOutput=.005
  wires:
  In1/1 -> Out1/1
